simulink model "electromagnet_b"  (R2024a)
settings: Solver=VariableStepAuto  StartTime=0.0  StopTime=te  MaxStep=te/100  RelTol=1e-3
values from neighbouring files (symbols this model uses):
  w = [0.5 1 2]    [sim21_solution.m]
  x0 = [0 0]    [sim21_solution.m]
undefined symbols (not defined in the file or in its folder): A, lfe, mu0, mur, N, Psi
settings Model: Creator=ocean  LastModifiedBy=ocean

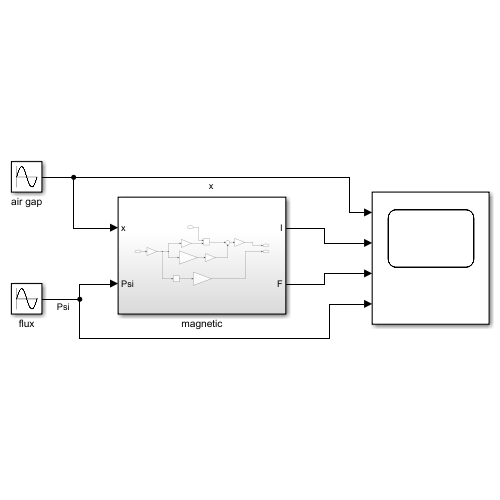
[thumbnail: Simulink's stored preview of the top-level diagram]
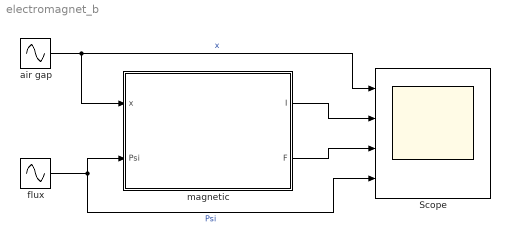
== system electromagnet_b ==
  Scope : Scope  NumInputPorts=4
  air gap : Sin  Amplitude=x0  Bias=x0  Frequency=w  SampleTime=0
  flux : Sin  Amplitude=Psi  Frequency=w  Phase=pi/2  SampleTime=0
  magnetic : Subsystem
  wires:
  air gap/1 -> Scope/1, magnetic/1(x)  "x"
  flux/1 -> Scope/4, magnetic/2(Psi)  "Psi"
  magnetic/1(I) -> Scope/2
  magnetic/2(F) -> Scope/3

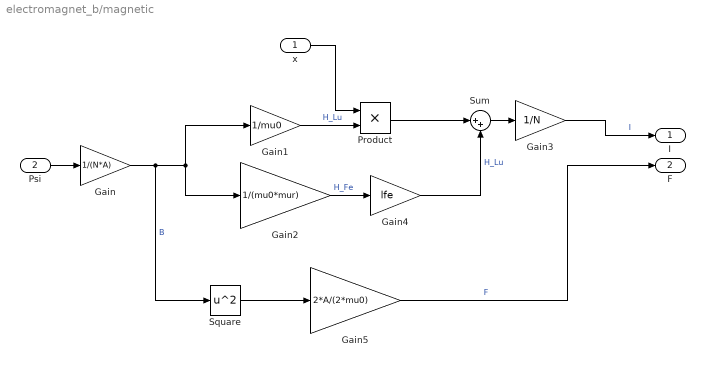
== system electromagnet_b/magnetic ==
  x : Inport
  Psi : Inport  Port=2
  Gain : Gain  Gain=1/(N*A)
  Gain1 : Gain  Gain=1/mu0
  Gain2 : Gain  Gain=1/(mu0*mur)
  Gain3 : Gain  Gain=1/N
  Gain4 : Gain  Gain=lfe
  Gain5 : Gain  Gain=2*A/(2*mu0)
  Product : Product
  Square : Math  Operator=square
  Sum : Sum  Inputs=|++
  I : Outport
  F : Outport  Port=2
  wires:
  Product/1 -> Sum/1
  Square/1 -> Gain5/1
  Gain/1 -> Square/1, Gain1/1, Gain2/1  "B"
  Gain4/1 -> Sum/2  "H_Lu"
  Gain2/1 -> Gain4/1  "H_Fe"
  Gain1/1 -> Product/2  "H_Lu"
  Sum/1 -> Gain3/1
  Gain3/1 -> I/1  "I"
  x/1 -> Product/1
  Gain5/1 -> F/1  "F"
  Psi/1 -> Gain/1
